simulink model "microgrid"  (R2021b)
settings: Solver=ode23tb  StartTime=0.0  StopTime=1  FixedStep=5e-6  RelTol=1e-3  EnableMultiTasking=on
PreLoadFcn:
  | % ---- microgrid : PreLoadFcn -------------------------------------
  | % Loads every base-workspace parameter this model needs.
  | %   SolarPVMPPTBoostData.mlx : PV array, boost converter, MPPT controller
  | %   microgridParams.m        : bus, battery, grid, drain, droop  (struct mg)
  | try
  |     mgDir = fileparts(which('microgrid'));
  |     if ~isempty(mgDir) && ~contains([path pathsep], [mgDir pathsep])
  |         addpath(mgDir);
  |     end
  |     evalc('SolarPVMPPTBoostData');
  |     microgridParams;
  |     clear mgDir
  |     disp('microgrid: parameters loaded (SolarPVMPPTBoostData + microgridParams).');
  | catch mgErr
  |     warning('microgrid:paramLoadFailed', ...
  |             'Could not load model parameters: %s', mgErr.message);
  |     clear mgErr
  | end
values from neighbouring files (symbols this model uses):
  mg = evalin('base','mg')    [microgridCheck.m]    (also in microgridParams.m = struct(); microgridScenario.m)
undefined symbols (not defined in the file or in its folder): boostController, dcVoltage, Ion, Lithium, sensor, solarPanel, solarPlant
libraries: powerlib_extras x46, fl_lib x12, simulink x8, nesl_utility x8, spsSeriesRLCBranchLib x7, spsCurrentMeasurementLib x7, spsGroundLib x6, spsVoltageMeasurementLib x6, spsIGBTDiodeLib x4, spsVariableResistorLib x4, slpidlib x4, ee_lib x3
(part 1 of 3)
settings Model: Creator=Student  LastModifiedBy=Saad Khan
settings SolverCC: ZeroCrossAlgorithm=Adaptive  AlgebraicLoopSolver=TrustRegion
settings DataIOCC: LimitDataPoints=on  SaveFormat=Array  SignalLoggingSaveFormat=ModelDataLogs  ReturnWorkspaceOutputs=off
settings OptimizationCC: ExpressionDepthLimit=2147483647  LifeSpan=inf
settings DebuggingCC: UnderspecifiedInitializationDetection=Classic  MergeDetectMultiDrivingBlocksExec=none  SolverPrmCheckMsg=warning  FcnCallInpInsideContextMsg=warning  StateNameClashWarn=warning  SFUnexpectedBacktrackingDiag=warning  SFNoUnconditionalDefaultTransitionDiag=warning  SFExecutionAtInitializationDiag=none  ArithmeticOperatorsInVariantConditions=warning
settings HardwareCC: ProdBitPerPointer=32  ProdBitPerSizeT=32  ProdBitPerPtrDiffT=32  ProdLargestAtomicFloat=None  ProdIntDivRoundTo=Undefined  ProdEndianess=Unspecified  ProdWordSize=32  ProdHWDeviceType=32-bit Generic
settings ModelReferenceCC: EnableRefExpFcnMdlSchedulingChecks=off  PropagateSignalLabelsOutOfModel=off
settings SFSimCC: SimUseLocalCustomCode=off  CustomCodeUndefinedFunction=UseInterfaceOnly
settings RTWCC: RTWUseLocalCustomCode=off  DLArmComputeVersion=20.02.1
settings CodeAppCC: StateflowObjectComments=on
settings GRTTargetCC: TargetLangStandard=C89/C90 (ANSI)  CombineOutputUpdateFcns=off  GRTInterface=on
settings ConfigComp: CovMetricSettings=dw  CovSaveCumulativeToWorkspaceVar=on  CovSaveSingleToWorkspaceVar=on  CovExternalEMLEnable=off
settings SimscapeCC: SimscapeNormalizeSystem=off

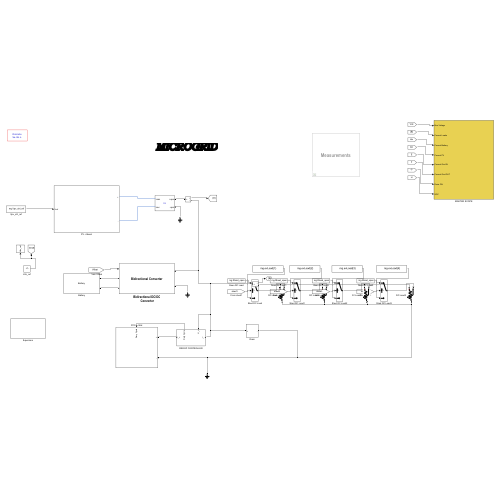
[thumbnail: Simulink's stored preview of the top-level diagram]
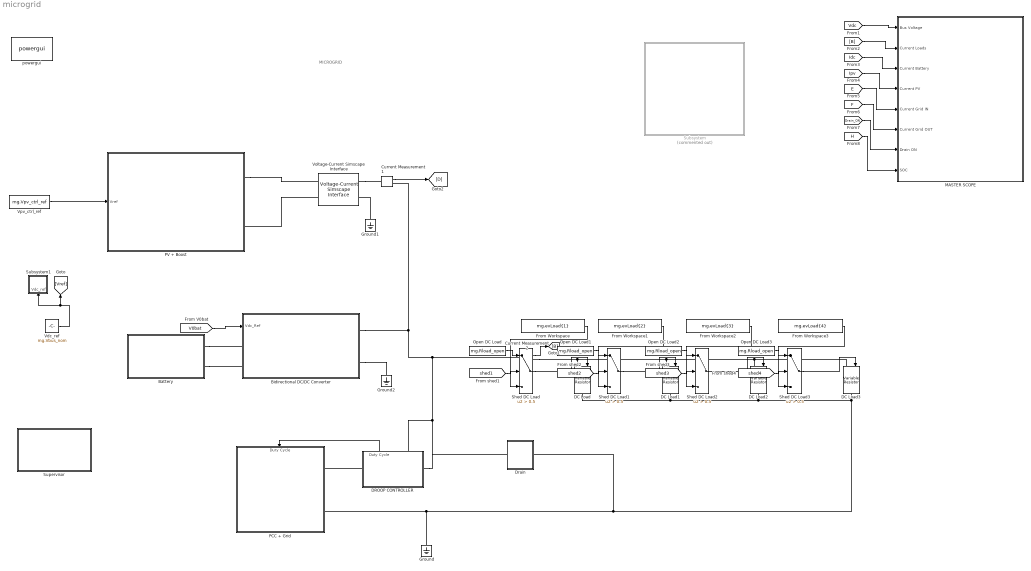
== system microgrid ==
  note: MICROGRID
  Battery : Subsystem
      mask Display:
      | %image(imread('Battery.bmp'))
      | disp('Battery');
  Bidirectional DC/DC Converter : Subsystem
      mask Display: disp('Bidirectional Converter')
  Current Measurement1 : spsCurrentMeasurementLib/Current Measurement  PhasorSimulation=off  OutputType=Complex  PSBequivalent=0
  Current Measurement2 : spsCurrentMeasurementLib/Current Measurement  PhasorSimulation=off  OutputType=Complex  PSBequivalent=0
  DC Load{,1..3} (4 alike) : spsVariableResistorLib/Variable Resistor  Rabsmin=1e-3
      settings: SourceProductBaseCode=PS
  DROOP CONTROLLER : Subsystem
      settings: PortSchema="{\"entries\":[{\"content\":{\"sides\":[{\"content\":{\"connectorIds\":[\"LConn1\"]},\"type\":\"ConnectorPlacement.EquallySpacedRectSide\",\"uuid\":\"2b7abaaf-3c10-498f-b261-e88602c8f41c\"},{\"content\":{\"connectorIds\":[\"RConn1\"],\"side\":\"RIGHT\"},\"type\":\"ConnectorPlacement.EquallySpacedRectSide\",\"uuid\":\"71817c43-ea35-4733-8571-129222f61f00\"},{\"content\":{\"connectorIds\":[\"Out1\",\"LConn2\"],\"side\":\"TOP\"},\"type\":\"ConnectorPlacement.EquallySpacedRectSide\",\"uuid\":\"db48e4ed-dd68-4965-9d82-541b8d604782\"},{\"content\":{\"connectorIds\":[],\"side\":\"BOTTOM\"},\"type\":\"ConnectorPlacement.EquallySpacedRectSide\",\"uuid\":\"50c4439a-898e-4973-8234-14cd96d1453b\"}]},\"type\":\"ConnectorPlacement.EquallySpacedConnector\",\"uuid\":\"1de87e89-706d-458a-94f9-225c5d9d3369\"}],\"packageUris\":[\"http://schema.mathworks.com/mf0/Connector/R2020b\"],\"version\":\"1.0\"}"
  Drain : Subsystem
  From Workspace : FromWorkspace  VariableName=mg.evLoad{1}
  From Workspace1 : FromWorkspace  VariableName=mg.evLoad{2}
  From Workspace2 : FromWorkspace  VariableName=mg.evLoad{3}
  From Workspace3 : FromWorkspace  VariableName=mg.evLoad{4}
  Ground : spsGroundLib/Ground  LConnTagsString=a
  Ground1 : spsGroundLib/Ground  LConnTagsString=a
  Ground2 : spsGroundLib/Ground  LConnTagsString=a
  MASTER SCOPE : Subsystem
  Open DC Load{,1..3} (4 alike) : Constant  Value=mg.Rload_open
  PCC + Grid : Subsystem
      settings: PortSchema="{\"entries\":[{\"content\":{\"sides\":[{\"content\":{\"connectorIds\":[\"LConn1\",\"LConn2\"]},\"type\":\"ConnectorPlacement.EquallySpacedRectSide\",\"uuid\":\"29bea7bc-953f-43d2-87dc-a51f4d1b9249\"},{\"content\":{\"connectorIds\":[],\"side\":\"RIGHT\"},\"type\":\"ConnectorPlacement.EquallySpacedRectSide\",\"uuid\":\"160e404e-4ddb-4454-97d5-9208db6d39a0\"},{\"content\":{\"connectorIds\":[\"In1\"],\"side\":\"TOP\"},\"type\":\"ConnectorPlacement.EquallySpacedRectSide\",\"uuid\":\"154aa630-8823-44c2-b2f2-ecc7273bc090\"}]},\"type\":\"ConnectorPlacement.EquallySpacedConnector\",\"uuid\":\"83e0acdf-9839-4104-a0b3-bfd87becac1e\"}],\"packageUris\":[\"http://schema.mathworks.com/mf0/Connector/R2020b\"],\"version\":\"1.0\"}"
  PV + Boost : Subsystem
  Shed DC Load{,1..3} (4 alike) : Switch  Criteria=u2 > Threshold  Threshold=0.5
  Subsystem : Subsystem  Commented=on
      mask Display: disp('Measurements')
  Subsystem1 : Subsystem
  Supervisor : Subsystem
  Vdc_ref : Constant  Value=mg.Vbus_nom
  Voltage-Current Simscape Interface : spsVoltageCurrentSimscapeInterfaceLib/Voltage-Current Simscape Interface  DFT=off  Fmode=Unit delay (discrete)  T=1e-6  Ts=-1  i0=0  v0=mg.Vbus_nom  Sd=Specialized Power Systems side  Measurements=off
      settings: SourceProductBaseCode=PS
  Vpv_ctrl_ref : Constant  Value=mg.Vpv_ctrl_ref
  powergui : spspowerguiLib/powergui  Priority=1  SimulationMode=Discrete  SampleTime=5e-6  frequency=50  Iterations=50  frequencyindice=0  Pbase=100e6  ErrMax=1e-4  UnitsV=kV  UnitsW=MW  buscounter=0  FunctionMessages=off  echomessages=off  EnableUseOfTLC=off  CurrentSourceSwitches=off  DisableSnubberDevices=off  DisableRonSwitches=off  DisableVfSwitches=off  DisplayEquations=off  AutomaticDiscreteSolvers=off  SolverType=Tustin  Interpol=off  ExternalGateDelay=off  methode=off  Ts=0  x0status=blocks  SPID=off  SwTol=0  HookPort=off  NonlinearTolerance=1e-4  nMaxIteration=100  ContinueOnMaxIteration=off  RestoreLinks=warning  ResistiveCurrentMeasurement=off  Frange=[0:2:500]  Ylog=off  Xlog=on  ShowGrid=off  save=off  variable=ZData  structure=Vab_st  ZoomFFT=off  StartTime=7.5  cycles=4  DisplayStyle=1  fundamental=50  FreqAxis=off  MaxFrequency=50000  frequencyindicesteady=1  RmsSteady=1  display=off
  wires:
  Vdc_ref/1 -> [Vref], Subsystem1/1(Vdc_ref)
  [Vdc] -> MASTER SCOPE/1(Bus Voltage)
  [E] -> MASTER SCOPE/5(Current Grid IN)
  [B] -> MASTER SCOPE/2(Current Loads)
  [Idc] -> MASTER SCOPE/3(Current Battery)
  [Ipv] -> MASTER SCOPE/4(Current PV)
  [F] -> MASTER SCOPE/6(Current Grid OUT)
  [Drain_ON] -> MASTER SCOPE/7(Drain ON)
  [H] -> MASTER SCOPE/8(SOC)
  Current Measurement2/1 -> [B]
  Current Measurement1/1 -> [D]
  DROOP CONTROLLER/1(Duty Cycle) -> PCC + Grid/1(" Dury Cycle ")
  Vpv_ctrl_ref/1 -> PV + Boost/1(Vref)
  [V0bat] -> Bidirectional DC/DC Converter/1(Vdc_Ref)
  Open DC Load/1 -> Shed DC Load/1
  [shed1] -> Shed DC Load/2
  From Workspace/1 -> Shed DC Load/3
  Shed DC Load/1 -> DC Load/1
  Open DC Load1/1 -> Shed DC Load1/1
  [shed2] -> Shed DC Load1/2
  From Workspace1/1 -> Shed DC Load1/3
  Shed DC Load1/1 -> DC Load1/1
  Open DC Load2/1 -> Shed DC Load2/1
  [shed3] -> Shed DC Load2/2
  From Workspace2/1 -> Shed DC Load2/3
  Shed DC Load2/1 -> DC Load2/1
  Open DC Load3/1 -> Shed DC Load3/1
  [shed4] -> Shed DC Load3/2
  From Workspace3/1 -> Shed DC Load3/3
  Shed DC Load3/1 -> DC Load3/1
  connections:
  Battery/LConn1 -- Bidirectional DC/DC Converter/LConn1
  Battery/LConn2 -- Bidirectional DC/DC Converter/LConn2
  Voltage-Current Simscape Interface/RConn2 -- PV + Boost/RConn2
  PV + Boost/RConn1 -- Voltage-Current Simscape Interface/RConn1
  Current Measurement2/LConn1 -- DROOP CONTROLLER/RConn1 -- Drain/LConn1 -- DROOP CONTROLLER/LConn2 -- Bidirectional DC/DC Converter/RConn1 -- Current Measurement1/RConn1
  DC Load3/LConn1 -- Current Measurement2/RConn1 -- DC Load/LConn1 -- DC Load1/LConn1 -- DC Load2/LConn1
  DC Load2/RConn1 -- Drain/RConn1 -- PCC + Grid/LConn2 -- Ground/LConn1 -- DC Load3/RConn1 -- DC Load/RConn1 -- DC Load1/RConn1
  Ground1/LConn1 -- Voltage-Current Simscape Interface/LConn2
  DROOP CONTROLLER/LConn1 -- PCC + Grid/LConn1
  Voltage-Current Simscape Interface/LConn1 -- Current Measurement1/LConn1
  Bidirectional DC/DC Converter/RConn2 -- Ground2/LConn1

== system microgrid/Battery ==
  Battery : spsBatteryLib/Battery  BatType=Lithium-Ion  ShowTempParam=off  ThermalPreset=no  ShowAgeParam=off  NomV=mg.Vbat_nom  NomQ=mg.Qbat_Ah  SOC=mg.SOC0  Batt_Tr=1  PresetModel=on  MaxQ=600  MinV=300  FullV=465.5949  Dis_rate=260.8696  R=0.0066667  Normal_OP=542.6087  expZone="[432.1543      29.47826]"  current=[1.3 2.6 6.5]  Units=Time  Tci=20  NomT=20  T2=-30  MaxQ2=4.8  FullV2=7.1  Normal_OP2=5.655  expZone2="[6.58           1]"  Rca=0.6  ti=2000  Dp=0  Neq0=0  Tsim=1e6  Ta1=25  Qeol=5.4*0.9  Reol=0.013333*1.2  Char_age=[2.3478, 3]  Dis_age=[2.3478, 10]  N1=1500  N2=10500  N3=1000  N4=1400  Ta2=45  N5=950
  Bus Selector : BusSelector  OutputSignals=SOC (%),Current (A),Voltage (V)
  Ground : spsGroundLib/Ground  LConnTagsString=a
  LPF vq1 : powerlib_extras/Discrete  Control Blocks/Discrete 1st-Order Filter  FilterType=Lowpass  Tc=10e-3  Ts=5e-6  Initialize=off  Vac_Init=[0.8 -25 60]  Vdc_Init=0  PlotResponse=off  param1=[1 100 0.1]
      settings: SourceProductBaseCode=PS
  LPF vq2 : powerlib_extras/Discrete  Control Blocks/Discrete 1st-Order Filter  FilterType=Lowpass  Tc=10e-3  Ts=5e-6  Initialize=off  Vac_Init=[0.8 -25 60]  Vdc_Init=0  PlotResponse=off  param1=[1 100 0.1]
      settings: SourceProductBaseCode=PS
  SOC : Scope
  Subsystem1 : Subsystem
  Subsystem2 : Subsystem
  Subsystem5 : Subsystem
  Vbat : Scope
  + : PMIOPort  Side=Left
  - : PMIOPort  Port=2  Side=Left
  tag scope: H=global
  wires:
  Battery/1 -> Bus Selector/1
  Bus Selector/2 -> LPF vq1/1  "<Current (A)>"
  LPF vq1/1 -> Subsystem1/1(Ibat)
  Bus Selector/1 -> [H], SOC/1, Subsystem5/1(SOC)  "<SOC (%)>"
  Bus Selector/3 -> Vbat/1, LPF vq2/1  "<Voltage (V)>"
  LPF vq2/1 -> Subsystem2/1(Vbat)
  connections:
  -/RConn1 -- Ground/LConn1 -- Battery/LConn2
  Battery/LConn1 -- +/RConn1

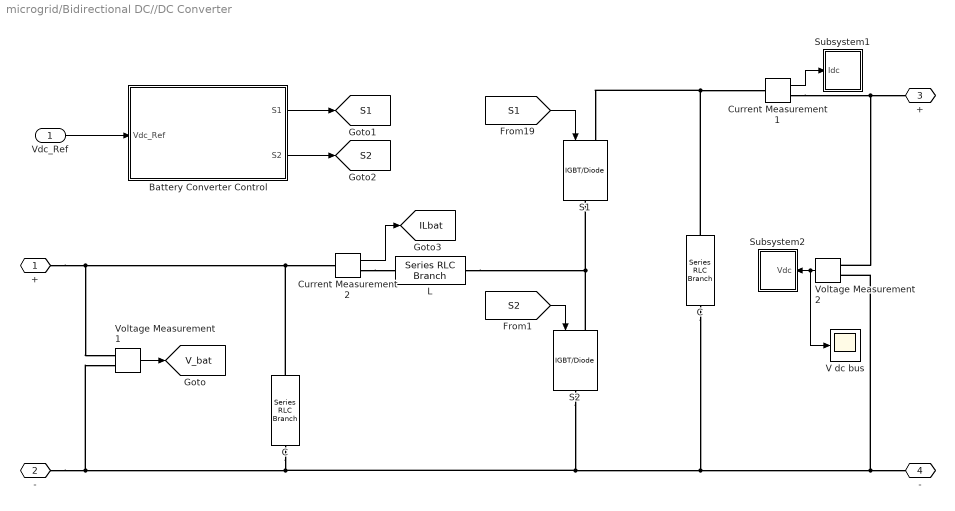
== system microgrid/Bidirectional DC//DC Converter ==
  Vdc_Ref : Inport
  Battery Converter Control : Subsystem
  C : spsSeriesRLCBranchLib/Series RLC Branch  LConnTagsString=__new0  RConnTagsString=__new0  BranchType=RC  Resistance=0.01  Inductance=1e-3  SetiL0=off  InitialCurrent=0  Capacitance=mg.Cbat_bus  Setx0=on  InitialVoltage=mg.Vbus_nom  Measurements=None
  "C " : spsSeriesRLCBranchLib/Series RLC Branch  LConnTagsString=__new0  RConnTagsString=__new0  BranchType=RC  Resistance=0.01  Inductance=1e-3  SetiL0=off  InitialCurrent=0  Capacitance=mg.Cbat  Setx0=on  InitialVoltage=mg.Vbat_C0  Measurements=None
  Current Measurement1 : spsCurrentMeasurementLib/Current Measurement  PhasorSimulation=off  OutputType=Complex  PSBequivalent=0
  Current Measurement2 : spsCurrentMeasurementLib/Current Measurement  PhasorSimulation=off  OutputType=Complex  PSBequivalent=0
  L : spsSeriesRLCBranchLib/Series RLC Branch  LConnTagsString=__new0  RConnTagsString=__new0  BranchType=L  Resistance=mg.Rbat_L  Inductance=mg.Lbat  SetiL0=on  InitialCurrent=0  Capacitance=1e-6  Setx0=off  InitialVoltage=0  Measurements=None
  "S1 " : spsIGBTDiodeLib/IGBT//Diode  Ron=mg.Ron  Rs=mg.Rsnub  Cs=inf  Measurements=off
  "S2 " : spsIGBTDiodeLib/IGBT//Diode  Ron=mg.Ron  Rs=mg.Rsnub  Cs=inf  Measurements=off
  Subsystem1 : Subsystem
  Subsystem2 : Subsystem
  V dc bus : Scope
  Voltage Measurement1 : spsVoltageMeasurementLib/Voltage Measurement  PhasorSimulation=off  OutputType=Complex  PSBequivalent=0
  Voltage Measurement2 : spsVoltageMeasurementLib/Voltage Measurement  PhasorSimulation=off  OutputType=Complex  PSBequivalent=0
  "+ " : PMIOPort  Side=Left
  "-  " : PMIOPort  Port=2  Side=Left
  + : PMIOPort  Port=3  Side=Right
  - : PMIOPort  Port=4  Side=Right
  tag scope: ILbat=global, S1=global, S2=global, V_bat=global
  wires:
  Voltage Measurement1/1 -> [V_bat]
  Current Measurement2/1 -> [ILbat]
  Battery Converter Control/1(S1) -> [S1]
  Battery Converter Control/2(S2) -> [S2]
  [S1] -> "S1 "/1
  [S2] -> "S2 "/1
  Voltage Measurement2/1 -> V dc bus/1, Subsystem2/1(Vdc)
  Current Measurement1/1 -> Subsystem1/1(Idc)
  Vdc_Ref/1 -> Battery Converter Control/1(Vdc_Ref)
  connections:
  "-  "/RConn1 -- Voltage Measurement1/LConn2 -- "C "/RConn1 -- "S2 "/RConn1 -- C/RConn1 -- -/RConn1 -- Voltage Measurement2/LConn2
  "S2 "/LConn1 -- "S1 "/RConn1 -- L/RConn1
  C/LConn1 -- "S1 "/LConn1 -- Current Measurement1/LConn1
  Current Measurement2/RConn1 -- L/LConn1
  "+ "/RConn1 -- Voltage Measurement1/LConn1 -- "C "/LConn1 -- Current Measurement2/LConn1
  Current Measurement1/RConn1 -- +/RConn1 -- Voltage Measurement2/LConn1

== system microgrid/DROOP CONTROLLER ==
  Current Measurement : spsCurrentMeasurementLib/Current Measurement  PhasorSimulation=off  OutputType=Complex  PSBequivalent=0
  Grid Droop : microgridLib/DC Droop Node  Rdroop=mg.Rdroop_grid  DB=mg.DB_grid  Tf=mg.Tf_droop  Imin=mg.Igrid_min  Imax=mg.Igrid_max  Vinit=mg.Vbus_nom
  Ground : spsGroundLib/Ground  LConnTagsString=a
  Igrid limit : simulink/Discontinuities/Saturation Dynamic  OutMin=[]  OutMax=[]  OutDataTypeStr=Inherit: Same as second input  OutDataType=fixdt(1, 16)  OutScaling=2^-10  DoSatur=off
  PID Controller : slpidlib/PID Controller  Controller=PI  Form=Parallel  TimeDomain=Continuous-time  UseExternalTs=off  SampleTime=-1  IntegratorMethod=Forward Euler  FilterMethod=Forward Euler  ControllerParametersSource=internal  P=mg.Kp_i_gdc  I=mg.Ki_i_gdc  D=0  UseFilter=on  N=100  TunerSelectOption=Transfer Function Based (PID Tuner App)  InitialConditionSource=internal  InitialConditionForIntegrator=mg.Dgdc_nom  InitialConditionForFilter=0  DifferentiatorICPrevScaledInput=0  ExternalReset=none  TrackingMode=off  Kt=1  LimitOutput=on  SatLimitsSource=internal  UpperSaturationLimit=1  LowerSaturationLimit=0  LinearizeAsGain=on  AntiWindupMode=clamping  Kb=1  POutMin=[]  POutMax=[]  IOutMin=[]  IOutMax=[]  DOutMin=[]  DOutMax=[]  NOutMin=[]  NOutMax=[]  SumOutMin=[]  SumOutMax=[]  SaturationOutMin=[]  SaturationOutMax=[]  PParamMin=[]  PParamMax=[]  IParamMin=[]  IParamMax=[]  DParamMin=[]  DParamMax=[]  NParamMin=[]  NParamMax=[]  KbParamMin=[]  KbParamMax=[]  KtParamMin=[]  KtParamMax=[]  KbOutMin=[]  KbOutMax=[]  KtOutMin=[]  KtOutMax=[]  IntegratorOutMin=[]  IntegratorOutMax=[]  FilterOutMin=[]  FilterOutMax=[]  SumI1OutMin=[]  SumI1OutMax=[]  SumI2OutMin=[]  SumI2OutMax=[]  SumI3OutMin=[]  SumI3OutMax=[]  SumI4OutMin=[]  SumI4OutMax=[]  SumDOutMin=[]  SumDOutMax=[]  DifferentiatorOutMin=[]  DifferentiatorOutMax=[]  FilterDiffOutCoefMin=[]  FilterDiffOutCoefMax=[]  ReciprocalOutMin=[]  ReciprocalOutMax=[]  SumDenOutMin=[]  SumDenOutMax=[]  SumNumOutMin=[]  SumNumOutMax=[]  DivideOutMin=[]  DivideOutMax=[]  UdiffTsProdOutMin=[]  UdiffTsProdOutMax=[]  NTsProdOutMin=[]  NTsProdOutMax=[]  UintegralTsProdOutMin=[]  UintegralTsProdOutMax=[]  UngainTsProdOutMin=[]  UngainTsProdOutMax=[]  FilterDenConstantOutDataTypeStr=Inherit: Inherit via back propagation  FilterDenConstantOutMin=[]  FilterDenConstantOutMax=[]  PCopyOutDataTypeStr=Inherit: Inherit via back propagation  PCopyOutMin=[]  PCopyOutMax=[]  NCopyOutDataTypeStr=Inherit: Inherit via back propagation  NCopyOutMin=[]  NCopyOutMax=[]  IntegratorContinuousStateAttributes=''  IntegratorStateMustResolveToSignalObject=off  IntegratorRTWStateStorageClass=Auto  FilterContinuousStateAttributes=''  FilterStateMustResolveToSignalObject=off  FilterRTWStateStorageClass=Auto  ParallelPVariant=InternalParameters  IdealPVariant=Disabled  IVariant=InternalParameters  DVariant=Disabled  IntegratorVariant=Continuous  SatVariant=Enabled  AWVariant=ContClampingParallel  PCopyVariant=Disabled  TRVariant=Disabled  FdbkBlocksVariant=Forward  IdealPFdbkVariant=Disabled  SatFdbkVariant=Disabled  DerivativeFilterVariant=Disabled  NVariant=Disabled  NCopyVariant=Disabled_SignalSpec  FilterICVariant=Disabled  IntegratorICVariant=InternalICs  ExternalResetVariant=Disabled  TRSumVariant=Passthrough  SumFdbkVariant=Disabled  SumVariant=Sum_PI  TsampFilterVariant=InternalTs  TsampNgainVariant=Passthrough  TsampIntegralVariant=Passthrough  ExternalSaturationOutDataTypeStr=Inherit: Same as second input
  Subtract1 : Sum  Inputs=+-
  Voltage Measurement : spsVoltageMeasurementLib/Voltage Measurement  PhasorSimulation=off  OutputType=Complex  PSBequivalent=0
  log Igrid ref : ToWorkspace  VariableName=Igrid_ref  SampleTime=-1
      settings: Decimation=20
  I_+ : PMIOPort  Side=Left
  U_+ : PMIOPort  Port=2  Side=Left
  I_- : PMIOPort  Port=3  Side=Right
  Duty Cycle : Outport
  tag scope: F=global
  wires:
  Subtract1/1 -> PID Controller/1
  PID Controller/1 -> [F], Duty Cycle/1
  Current Measurement/1 -> Subtract1/2
  [V0grid] -> Grid Droop/1
  Voltage Measurement/1 -> Grid Droop/2
  [Igrid_hi] -> Igrid limit/1
  Grid Droop/1 -> Igrid limit/2
  [Igrid_lo] -> Igrid limit/3
  Igrid limit/1 -> Subtract1/1, log Igrid ref/1
  connections:
  I_-/RConn1 -- Current Measurement/RConn1
  Voltage Measurement/LConn1 -- U_+/RConn1
  I_+/RConn1 -- Current Measurement/LConn1
  Ground/LConn1 -- Voltage Measurement/LConn2

== system microgrid/Drain ==
  Current Measurement1 : spsCurrentMeasurementLib/Current Measurement  PhasorSimulation=off  OutputType=Complex  PSBequivalent=0
  Drain hysteresis : Relay  OnSwitchValue=mg.Vdrain_on  OffSwitchValue=mg.Vdrain_off
  Ground : spsGroundLib/Ground  LConnTagsString=a
  Ideal Switch : spsIdealSwitchLib/Ideal Switch  Ron=mg.Rdrain_on  Lon=0  IC=0  Rs=9999999  Cs=inf  Measurements=off
  Idrain filt term : Terminator
  Series RLC Branch : spsSeriesRLCBranchLib/Series RLC Branch  LConnTagsString=__new0  RConnTagsString=__new0  BranchType=R  Resistance=mg.Rdrain  Inductance=1e-3  SetiL0=off  InitialCurrent=0  Capacitance=1e-6  Setx0=off  InitialVoltage=0  Measurements=None
  Transfer Fcn : TransferFcn  Denominator=[1 1]
  Voltage Measurement : spsVoltageMeasurementLib/Voltage Measurement  PhasorSimulation=off  OutputType=Complex  PSBequivalent=0
  + : PMIOPort  Side=Left
  - : PMIOPort  Port=2  Side=Right
  tag scope: Drain_ON=global
  wires:
  Current Measurement1/1 -> Transfer Fcn/1
  Transfer Fcn/1 -> Idrain filt term/1
  Voltage Measurement/1 -> Drain hysteresis/1
  Drain hysteresis/1 -> Ideal Switch/1, [Drain_ON]
  connections:
  Ideal Switch/LConn1 -- Voltage Measurement/LConn1 -- +/RConn1
  Series RLC Branch/RConn1 -- -/RConn1
  Ground/LConn1 -- Voltage Measurement/LConn2
  Current Measurement1/LConn1 -- Ideal Switch/RConn1
  Current Measurement1/RConn1 -- Series RLC Branch/LConn1

== system microgrid/MASTER SCOPE ==
  Bus Voltage : Inport
  Current Loads : Inport  Port=2
  Current Battery : Inport  Port=3
  Current PV : Inport  Port=4
  Current Grid IN : Inport  Port=5
  Current Grid OUT : Inport  Port=6
  Drain ON : Inport  Port=7
  SOC : Inport  Port=8
  MASTER SCOPE : Scope  NumInputPorts=8
  wires:
  Bus Voltage/1 -> MASTER SCOPE/1
  Current Loads/1 -> MASTER SCOPE/2
  Current Battery/1 -> MASTER SCOPE/3
  Current PV/1 -> MASTER SCOPE/4
  Current Grid IN/1 -> MASTER SCOPE/5
  Current Grid OUT/1 -> MASTER SCOPE/6
  Drain ON/1 -> MASTER SCOPE/7
  SOC/1 -> MASTER SCOPE/8

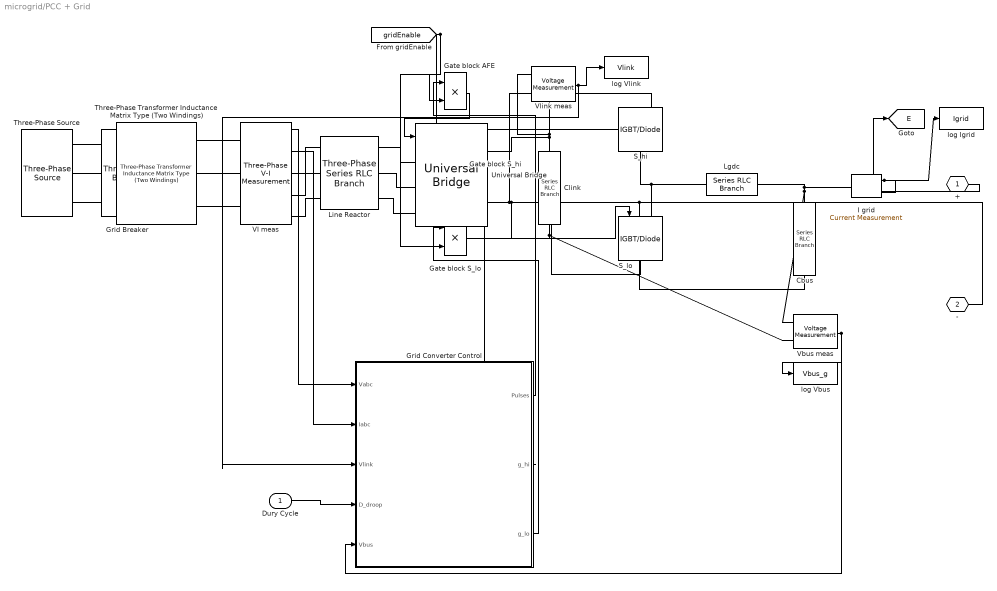
== system microgrid/PCC + Grid ==
  " Dury Cycle " : Inport
  Cbus : spsSeriesRLCBranchLib/Series RLC Branch  LConnTagsString=__new0  RConnTagsString=__new0  BranchType=RC  Resistance=mg.Resr  Inductance=1e-3  SetiL0=off  InitialCurrent=0  Capacitance=mg.Cgdc_bus  Setx0=on  InitialVoltage=mg.Vbus_nom  Measurements=None
  Clink : spsSeriesRLCBranchLib/Series RLC Branch  LConnTagsString=__new0  RConnTagsString=__new0  BranchType=C  Resistance=1  Inductance=1e-3  SetiL0=off  InitialCurrent=0  Capacitance=mg.Clink  Setx0=on  InitialVoltage=mg.Vlink_ref  Measurements=None
  Gate block AFE : Product
  Gate block S_hi : Product
  Gate block S_lo : Product
  Grid Breaker : spsThreePhaseBreakerLib/Three-Phase Breaker  InitialState=closed  SwitchA=on  SwitchB=on  SwitchC=on  SwitchTimes=[mg.t_island mg.t_reconnect]  External=off  BreakerResistance=mg.Ron  SnubberResistance=mg.Rsnub  SnubberCapacitance=inf  Measurements=None
  Grid Converter Control : Subsystem
  I grid : spsCurrentMeasurementLib/Current Measurement  PhasorSimulation=off  OutputType=Complex  PSBequivalent=0
  Lgdc : spsSeriesRLCBranchLib/Series RLC Branch  LConnTagsString=__new0  RConnTagsString=__new0  BranchType=L  Resistance=mg.Rgdc  Inductance=mg.Lgdc  SetiL0=off  InitialCurrent=0  Capacitance=1e-6  Setx0=off  InitialVoltage=0  Measurements=None
  Line Reactor : spsThreePhaseSeriesRLCBranchLib/Three-Phase Series RLC Branch  LConnTagsString=A|B|C  RConnTagsString=A|B|C  BranchType=RL  Resistance=mg.Rgrid  Inductance=mg.Lgrid  Capacitance=1e-6  Measurements=None
  S_hi : spsIGBTDiodeLib/IGBT//Diode  Ron=mg.Ron  Rs=mg.Rsnub  Cs=mg.Csnub  Measurements=off
  S_lo : spsIGBTDiodeLib/IGBT//Diode  Ron=mg.Ron  Rs=mg.Rsnub  Cs=mg.Csnub  Measurements=off
  Three-Phase Source : spsThreePhaseSourceLib/Three-Phase Source  InternalConnection=Yg  VoltagePhases=off  Voltage=mg.Vgrid_LL  PhaseAngle=0  Voltage_phases=[25e3 25e3 25e3]/sqrt(3)  PhaseAngles_phases=[0 -120 +120]  Frequency=mg.fgrid  NonIdealSource=on  SpecifyImpedance=off  Resistance=0.8929  Inductance=16.58e-3  ShortCircuitLevel=100e6  BaseVoltage=25e3  XRratio=7  BusType=swing  Pref=10e3  Qref=0  Prefabc=[10e3, 10e3, 10e3]  Qrefabc=[0, 0, 0]  Qmin=-inf  Qmax=inf
  Three-Phase Transformer Inductance Matrix Type (Two Windings) : spsThreePhaseTransformerInductanceMatrixTypeTwoWindingsLib/Three-Phase Transformer Inductance Matrix Type (Two Windings)  CoreType=Three-limb or five-limb core  Winding1Connection=Yg  Winding2Connection=Y  AutoTransformer=off  Measurements=None  NominalPower=[800e3, 50]  VLLnom=[25000, 800]  WindingResistances=[0.01, 0.01]  NoLoadIexcPos=2  NoLoadPlossPos=1000  ShortCircuitReactancePos=0.06  ShortCircuitReactancePosAuto=0.06  NoLoadIexcZero=2  NoLoadPlossZero=1500  ShortCircuitReactanceZero=0.03  ShortCircuitReactanceZeroAuto=0.03
      settings: SourceProductBaseCode=PS
  Universal Bridge : spsUniversalBridgeLib/Universal Bridge  Arms=3  SnubberResistance=mg.Rsnub  SnubberCapacitance=mg.Csnub  Device=IGBT / Diodes  Ron=mg.Ron  Lon=0  ForwardVoltages="[  0  0  ]"  ForwardVoltage=0  GTOparameters=[ 10e-6 , 20e-6 ]  IGBTparameters=[ 1e-6 , 2e-6 ]  Measurements=None  Measurements_2=None  converterType=Rectifier
  VI meas : spsThreePhaseVIMeasurementLib/Three-Phase V-I Measurement  VoltageMeasurement=phase-to-ground  SetLabelV=off  LabelV=Vabc  Vpu=off  VpuLL=off  CurrentMeasurement=yes  SetLabelI=off  LabelI=Iabc  Ipu=off  Pbase=100e6  Vbase=500e3  OutputType=Complex  PhasorSimulation=off  PSBequivalent=0
  Vbus meas : spsVoltageMeasurementLib/Voltage Measurement  PhasorSimulation=off  OutputType=Complex  PSBequivalent=0
  Vlink meas : spsVoltageMeasurementLib/Voltage Measurement  PhasorSimulation=off  OutputType=Complex  PSBequivalent=0
  log Igrid : ToWorkspace  VariableName=Igrid  SampleTime=-1
      settings: Decimation=20
  log Vbus : ToWorkspace  VariableName=Vbus_g  SampleTime=-1
      settings: Decimation=20
  log Vlink : ToWorkspace  VariableName=Vlink  SampleTime=-1
      settings: Decimation=20
  + : PMIOPort  Side=Left
  - : PMIOPort  Port=2  Side=Left
  tag scope: E=global
  wires:
  I grid/1 -> [E], log Igrid/1
  VI meas/1 -> Grid Converter Control/1(Vabc)
  VI meas/2 -> Grid Converter Control/2(Iabc)
  Vlink meas/1 -> Grid Converter Control/3(Vlink), log Vlink/1
  " Dury Cycle "/1 -> Grid Converter Control/4(D_droop)
  Vbus meas/1 -> Grid Converter Control/5(Vbus), log Vbus/1
  Grid Converter Control/1(Pulses) -> Gate block AFE/1
  [gridEnable] -> Gate block AFE/2, Gate block S_hi/2, Gate block S_lo/2
  Gate block AFE/1 -> Universal Bridge/1
  Grid Converter Control/2(g_hi) -> Gate block S_hi/1
  Gate block S_hi/1 -> S_hi/1
  Grid Converter Control/3(g_lo) -> Gate block S_lo/1
  Gate block S_lo/1 -> S_lo/1
  connections:
  Three-Phase Transformer Inductance Matrix Type (Two Windings)/RConn1 -- VI meas/LConn1
  Three-Phase Transformer Inductance Matrix Type (Two Windings)/RConn2 -- VI meas/LConn2
  Three-Phase Transformer Inductance Matrix Type (Two Windings)/RConn3 -- VI meas/LConn3
  VI meas/RConn1 -- Line Reactor/LConn1
  VI meas/RConn2 -- Line Reactor/LConn2
  VI meas/RConn3 -- Line Reactor/LConn3
  Line Reactor/RConn1 -- Universal Bridge/LConn1
  Line Reactor/RConn2 -- Universal Bridge/LConn2
  Line Reactor/RConn3 -- Universal Bridge/LConn3
  Universal Bridge/RConn1 -- S_hi/LConn1 -- Vlink meas/LConn1 -- Clink/LConn1
  Universal Bridge/RConn2 -- -/RConn1 -- Cbus/RConn1 -- S_lo/RConn1 -- Clink/RConn1 -- Vbus meas/LConn2 -- Vlink meas/LConn2
  S_lo/LConn1 -- S_hi/RConn1 -- Lgdc/LConn1
  Lgdc/RConn1 -- I grid/LConn1 -- Cbus/LConn1 -- Vbus meas/LConn1
  I grid/RConn1 -- +/RConn1
  Three-Phase Source/RConn1 -- Grid Breaker/LConn1
  Grid Breaker/RConn1 -- Three-Phase Transformer Inductance Matrix Type (Two Windings)/LConn1
  Three-Phase Source/RConn2 -- Grid Breaker/LConn2
  Grid Breaker/RConn2 -- Three-Phase Transformer Inductance Matrix Type (Two Windings)/LConn2
  Three-Phase Source/RConn3 -- Grid Breaker/LConn3
  Grid Breaker/RConn3 -- Three-Phase Transformer Inductance Matrix Type (Two Windings)/LConn3

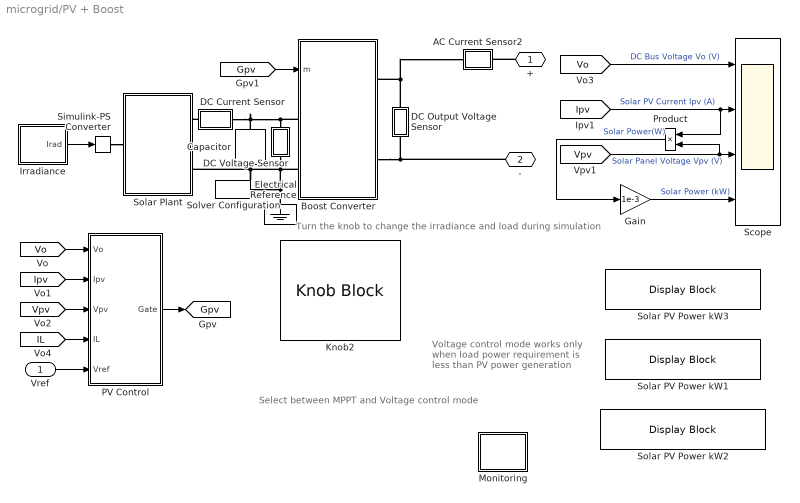
== system microgrid/PV + Boost ==
  note: Voltage control mode works only when load power requirement is less than PV power generation
  note: Select between MPPT and Voltage control mode
  note: Turn the knob to change the irradiance and load during simulation
  Vref : Inport
  AC Current Sensor2 : Subsystem
      mask Display: disp('i');
  Boost Converter : Subsystem  VariantControl=boostCircuit == 1
  Capacitor : fl_lib/Electrical/Electrical Elements/Capacitor  c=boost.inputCapacitor F  r=1e-6 Ohm  g=0 1/Ohm  i_specify=off  i_priority=None  i=0 A  i_nominal_specify=off  i_nominal_unit=A  i_nominal_value=1  v_specify=off  v_priority=None  v=solarPlant.startMPPTValue V  v_nominal_specify=off  v_nominal_unit=V  v_nominal_value=1  vc_specify=on  vc_priority=High  vc=solarPlant.startMPPTValue V  vc_nominal_specify=off  vc_nominal_unit=V  vc_nominal_value=1
  DC Current Sensor : Subsystem
      mask Display: disp('i')
  DC Output Voltage Sensor : Subsystem
      mask Display: disp('v')
  DC Voltage Sensor : Subsystem
      mask Display: disp('v');
  Electrical Reference : fl_lib/Electrical/Electrical Elements/Electrical Reference
  Gain : Gain  Gain=1e-3
  Irradiance : Subsystem
  Knob2 : KnobBlock  ScaleMin=150  ScaleMax=1000
  Monitoring : Subsystem
  PV Control : Subsystem
  Product : Product
  Scope : Scope  NumInputPorts=4
  Simulink-PS Converter : nesl_utility/Simulink-PS Converter  PhysicalDomain=network_engine_domain  SubClassName=ps_input  LeftPortType=input  RightPortType=output  PseudoPeriodic=off  Frequencies=[]  NoiseDistribution=none  NoiseParameters=[]  Unit=1  AffineConversion=off  FilteringAndDerivatives=provide  SimscapeFilterOrder=1  InputFilterTimeConstant=0.001  UdotUserProvided=0
      settings: SourceProductBaseCode=PW,SS
  Solar PV Power kW1 : DisplayBlock  Format=short  Transparency=1
  Solar PV Power kW2 : DisplayBlock  Format=short  Transparency=1
  Solar PV Power kW3 : DisplayBlock  Format=short  Transparency=1
  Solar Plant : Subsystem
  Solver Configuration : nesl_utility/Solver Configuration  PhysicalDomain=network_engine_domain  SubClassName=solver  LeftPortType=input  RightPortType=generic  Tones=[]  Harmonics=[]  SimulateNoise=off  Profile=off  UseLocalSampling=off  EnableSwitchedLinearOptims=on  FrequencyDomain=off  UseCCode=off  RelTol=0.001  AbsTol=1e-06  MinStep=1e-09  ToWorkspace=off  RevertToSquareIcSolve=off  NumHomotopyIterations=100  PhasorMode=off  PhasorModeNumHarmonics=1  DoDC=off  ResidualTolerance=1e-9  UseLocalSolver=off  LocalSolverChoice=NE_BACKWARD_EULER_ADVANCER  LocalSolverSampleTime=1e-6  DoFixedCost=off  MaxNonlinIter=10  MaxModeIter=2  ComputeImpulses=off  ImpulseIterations=2  LinearAlgebra=auto  EquationFormulation=NE_TIME_EF  DelaysMemoryBudget=1024  AutomaticFiltering=on  FilteringTimeConstant=0.001  PartitionStorageMethod=AS_NEEDED  PartitionMemoryBudget=1024  PartitionMethod=FAST
      settings: SourceProductBaseCode=PW,SS
  + : PMIOPort  Side=Right
  - : PMIOPort  Port=2  Side=Right
  tag scope: Gpv=global
  wires:
  [IL] -> PV Control/4(IL)
  Irradiance/1(Irad) -> Simulink-PS Converter/1
  [Ipv] -> PV Control/2(Ipv)
  [Ipv] -> Product/1, Scope/2  "Solar PV Current Ipv (A)"
  PV Control/1(Gate) -> [Gpv]
  [Vo] -> PV Control/1(Vo)
  [Vpv] -> Product/2, Scope/3  "Solar Panel Voltage Vpv (V)"
  [Vpv] -> PV Control/3(Vpv)
  Product/1 -> Gain/1  "Solar Power(W)"
  [Vo] -> Scope/1  "DC Bus Voltage Vo (V)"
  [Gpv] -> Boost Converter/1(m)
  Gain/1 -> Scope/4  "Solar Power (kW)"
  Vref/1 -> PV Control/5(Vref)
  connections:
  Electrical Reference/LConn1 -- Solar Plant/RConn2 -- Capacitor/RConn1 -- Boost Converter/LConn2 -- DC Voltage Sensor/LConn1 -- Solver Configuration/RConn1
  Boost Converter/LConn1 -- DC Voltage Sensor/RConn1 -- DC Current Sensor/LConn1 -- Capacitor/LConn1
  DC Current Sensor/RConn1 -- Solar Plant/RConn1
  Boost Converter/RConn2 -- -/RConn1 -- DC Output Voltage Sensor/LConn1
  Simulink-PS Converter/RConn1 -- Solar Plant/LConn1
  +/RConn1 -- AC Current Sensor2/LConn1
  Boost Converter/RConn1 -- DC Output Voltage Sensor/RConn1 -- AC Current Sensor2/RConn1

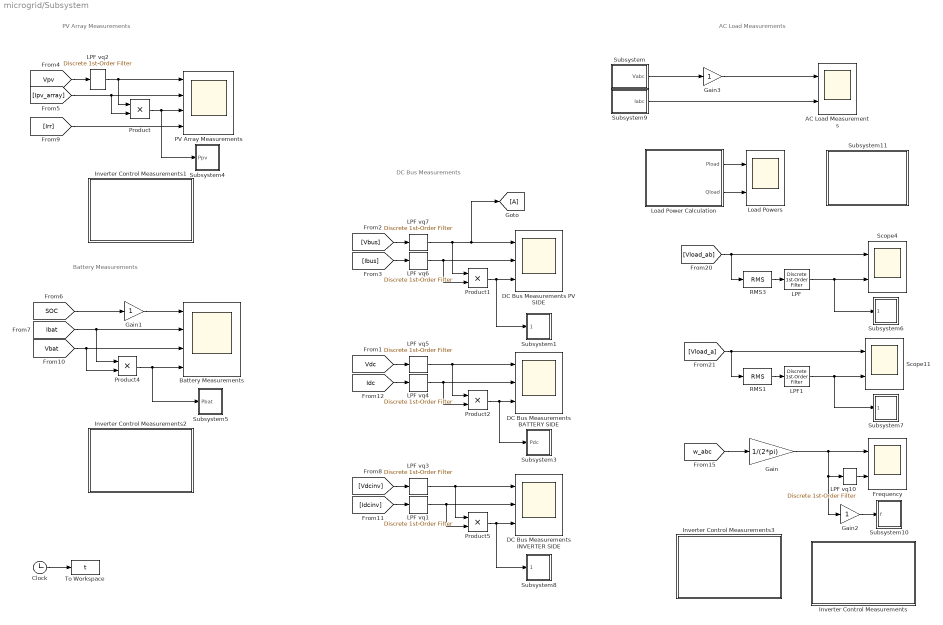
== system microgrid/Subsystem ==
  note: PV Array Measurements
  note: Battery Measurements
  note: DC Bus Measurements
  note: AC Load Measurements
  AC Load Measurements : Scope  NumInputPorts=2
  Battery Measurements : Scope  NumInputPorts=4
  Clock : Clock
  DC Bus Measurements BATTERY SIDE : Scope  NumInputPorts=3
  DC Bus Measurements INVERTER SIDE : Scope  NumInputPorts=3
  DC Bus Measurements PV SIDE : Scope  NumInputPorts=3
  Frequency : Scope  NumInputPorts=2
  Gain : Gain  Gain=1/(2*pi)
  Gain1 : Gain
  Gain2 : Gain
  Gain3 : Gain
  Inverter Control Measurements : Subsystem
      mask Display: disp('Inverter Control')
  Inverter Control Measurements1 : Subsystem
      mask Display: disp('Boost Converter Control')
  Inverter Control Measurements2 : Subsystem
      mask Display: disp('Bidirectional Converter Control')
  Inverter Control Measurements3 : Subsystem
      mask Display: disp('Frequency Measurement')
  LPF : powerlib_extras/Discrete  Control Blocks/Discrete 1st-Order Filter  FilterType=Lowpass  Tc=10e-3  Ts=5e-6  Initialize=off  Vac_Init=[0.8 -25 60]  Vdc_Init=0  PlotResponse=off  param1=[1 100 0.1]
      settings: SourceProductBaseCode=PS
  LPF vq{1..7,10} (8 alike) : powerlib_extras/Discrete  Control Blocks/Discrete 1st-Order Filter  FilterType=Lowpass  Tc=10e-3  Ts=5e-6  Initialize=off  Vac_Init=[0.8 -25 60]  Vdc_Init=0  PlotResponse=off  param1=[1 100 0.1]
      settings: SourceProductBaseCode=PS
  LPF1 : powerlib_extras/Discrete  Control Blocks/Discrete 1st-Order Filter  FilterType=Lowpass  Tc=10e-3  Ts=5e-6  Initialize=off  Vac_Init=[0.8 -25 60]  Vdc_Init=0  PlotResponse=off  param1=[1 100 0.1]
      settings: SourceProductBaseCode=PS
  Load Power Calculation : Subsystem
  Load Powers : Scope  NumInputPorts=2
  PV Array Measurements : Scope  NumInputPorts=4
  Product{,1..2,4..5} (5 alike) : Product  RndMeth=Zero
  RMS1 : powerlib_extras/Measurements/RMS  f1=60
      settings: SourceProductBaseCode=PS
  RMS3 : powerlib_extras/Measurements/RMS  f1=60
      settings: SourceProductBaseCode=PS
  Scope11 : Scope  NumInputPorts=2
  Scope4 : Scope  NumInputPorts=2
  Subsystem : Subsystem
  Subsystem1 : Subsystem
  Subsystem10 : Subsystem
  Subsystem11 : Subsystem
      mask Display: disp('Additional Load Meas.')
  Subsystem3 : Subsystem
  Subsystem4 : Subsystem
  Subsystem5 : Subsystem
  Subsystem6 : Subsystem
  Subsystem7 : Subsystem
  Subsystem8 : Subsystem
  Subsystem9 : Subsystem
  To Workspace : ToWorkspace  VariableName=t  SampleTime=5e-6
  wires:
  Product/1 -> PV Array Measurements/3, Subsystem4/1(Ppv)
  [Vpv] -> LPF vq2/1
  [Ipv_array] -> PV Array Measurements/2, Product/2
  [Irr] -> PV Array Measurements/4
  [SOC] -> Gain1/1
  [Ibat] -> Battery Measurements/2, Product4/1
  [Vbat] -> Battery Measurements/3, Product4/2
  Product4/1 -> Battery Measurements/4, Subsystem5/1(Pbat)
  [Vdc] -> LPF vq5/1
  [Idc] -> LPF vq4/1
  Product2/1 -> DC Bus Measurements BATTERY SIDE/3, Subsystem3/1(Pdc)
  Product1/1 -> DC Bus Measurements PV SIDE/3, Subsystem1/1(Pbus)
  [Vbus] -> LPF vq7/1
  [Ibus] -> LPF vq6/1
  Load Power Calculation/1(Pload) -> Load Powers/1
  Load Power Calculation/2(Qload) -> Load Powers/2
  [Vload_a] -> Scope11/1, RMS1/1
  RMS1/1 -> LPF1/1
  [Vload_ab] -> Scope4/1, RMS3/1
  RMS3/1 -> LPF/1
  LPF/1 -> Scope4/2, Subsystem6/1(Vab_rms)
  LPF1/1 -> Scope11/2, Subsystem7/1(Va_rms)
  Clock/1 -> To Workspace/1
  Product5/1 -> Subsystem8/1(Pdcinv), DC Bus Measurements INVERTER SIDE/3
  [Vdcinv] -> LPF vq3/1
  [Idcinv] -> LPF vq1/1
  LPF vq2/1 -> PV Array Measurements/1, Product/1
  LPF vq1/1 -> DC Bus Measurements INVERTER SIDE/2, Product5/2
  LPF vq3/1 -> DC Bus Measurements INVERTER SIDE/1, Product5/1
  LPF vq4/1 -> Product2/2, DC Bus Measurements BATTERY SIDE/2
  LPF vq5/1 -> Product2/1, DC Bus Measurements BATTERY SIDE/1
  LPF vq6/1 -> DC Bus Measurements PV SIDE/2, Product1/2
  LPF vq7/1 -> [A], DC Bus Measurements PV SIDE/1, Product1/1
  [w_abc] -> Gain/1
  Gain/1 -> Frequency/1, LPF vq10/1, Gain2/1
  LPF vq10/1 -> Frequency/2
  Subsystem9/1(Iabc) -> AC Load Measurements/2
  Subsystem/1(Vabc) -> Gain3/1
  Gain1/1 -> Battery Measurements/1
  Gain2/1 -> Subsystem10/1(f)
  Gain3/1 -> AC Load Measurements/1

== system microgrid/Subsystem1 ==
  Vdc_ref : Inport
  LPF vq6 : powerlib_extras/Discrete  Control Blocks/Discrete 1st-Order Filter  FilterType=Lowpass  Tc=10e-3  Ts=5e-6  Initialize=on  Vac_Init=[0.8 -25 60]  Vdc_Init=mg.Vbus_nom  PlotResponse=off  param1=[1 100 0.1]
      settings: SourceProductBaseCode=PS
  To Workspace1 : ToWorkspace  VariableName=Vdc_ref  SampleTime=-1
  tag scope: Vdc_ref=global
  wires:
  Vdc_ref/1 -> LPF vq6/1
  LPF vq6/1 -> [Vdc_ref], To Workspace1/1

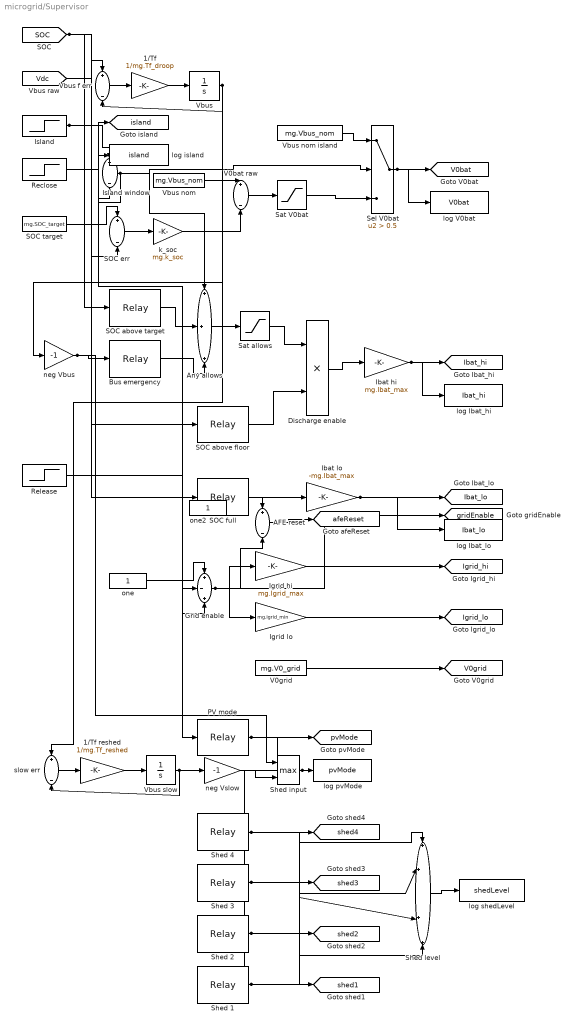
== system microgrid/Supervisor ==
  1/Tf : Gain  Gain=1/mg.Tf_droop
  1/Tf reshed : Gain  Gain=1/mg.Tf_reshed
  AFE reset : Sum  Inputs=+-
  Any allows : Sum  Inputs=+++
  Bus emergency : Relay  OnSwitchValue=-mg.Vbus_emerg  OffSwitchValue=-mg.Vbus_emerg_off
  Discharge enable : Product
  Grid enable : Sum  Inputs=+-+
  Ibat hi : Gain  Gain=mg.Ibat_max
  Ibat lo : Gain  Gain=-mg.Ibat_max
  Igrid hi : Gain  Gain=mg.Igrid_max
  Igrid lo : Gain  Gain=mg.Igrid_min
  Island : Step  Time=mg.t_island  SampleTime=0
  Island window : Sum  Inputs=+-
  PV mode : Relay  OnSwitchValue=mg.Vpv_ctrl_on  OffSwitchValue=mg.Vpv_ctrl_off  OnOutputValue=0  OffOutputValue=1
  Reclose : Step  Time=mg.t_reconnect  SampleTime=0
  Release : Step  Time=mg.t_reconnect+mg.t_resync  SampleTime=0
  SOC above floor : Relay  OnSwitchValue=mg.SOC_min+mg.SOC_hyst  OffSwitchValue=mg.SOC_min
  SOC above target : Relay  OnSwitchValue=mg.SOC_target+mg.SOC_hyst/2  OffSwitchValue=mg.SOC_target-mg.SOC_hyst/2
  SOC err : Sum  Inputs=+-
  SOC full : Relay  OnSwitchValue=mg.SOC_max  OffSwitchValue=mg.SOC_max-mg.SOC_hyst  OnOutputValue=0  OffOutputValue=1
  SOC target : Constant  Value=mg.SOC_target
  Sat V0bat : Saturate  UpperLimit=mg.V0bat_max  LowerLimit=mg.V0bat_min
  Sat allows : Saturate  UpperLimit=1  LowerLimit=0
  Sel V0bat : Switch  Criteria=u2 > Threshold  Threshold=0.5
  Shed 1 : Relay  OnSwitchValue=-mg.Vshed(4)  OffSwitchValue=-mg.Vshed_rst(4)
  Shed 2 : Relay  OnSwitchValue=-mg.Vshed(3)  OffSwitchValue=-mg.Vshed_rst(3)
  Shed 3 : Relay  OnSwitchValue=-mg.Vshed(2)  OffSwitchValue=-mg.Vshed_rst(2)
  Shed 4 : Relay  OnSwitchValue=-mg.Vshed(1)  OffSwitchValue=-mg.Vshed_rst(1)
  Shed input : MinMax  Function=max  Inputs=2
  Shed level : Sum  Inputs=++++
  V0bat raw : Sum  Inputs=+-
  V0grid : Constant  Value=mg.V0_grid
  Vbus : Integrator  InitialCondition=mg.Vbus_nom
  Vbus f err : Sum  Inputs=+-
  Vbus nom : Constant  Value=mg.Vbus_nom
  Vbus nom island : Constant  Value=mg.Vbus_nom
  Vbus slow : Integrator  InitialCondition=mg.Vbus_nom
  k_soc : Gain  Gain=mg.k_soc
  log Ibat_hi : ToWorkspace  VariableName=Ibat_hi  SaveFormat=Structure With Time  SampleTime=-1
      settings: Decimation=20
  log Ibat_lo : ToWorkspace  VariableName=Ibat_lo  SaveFormat=Structure With Time  SampleTime=-1
      settings: Decimation=20
  log V0bat : ToWorkspace  VariableName=V0bat  SaveFormat=Structure With Time  SampleTime=-1
      settings: Decimation=20
  log island : ToWorkspace  VariableName=island  SaveFormat=Structure With Time  SampleTime=-1
      settings: Decimation=20
  log pvMode : ToWorkspace  VariableName=pvMode  SaveFormat=Structure With Time  SampleTime=-1
      settings: Decimation=20
  log shedLevel : ToWorkspace  VariableName=shedLevel  SaveFormat=Structure With Time  SampleTime=-1
      settings: Decimation=20
  neg Vbus : Gain  Gain=-1
  neg Vslow : Gain  Gain=-1
  one : Constant
  one2 : Constant
  slow err : Sum  Inputs=+-
  tag scope: Ibat_hi=global, Ibat_lo=global, Igrid_hi=global, Igrid_lo=global, V0bat=global, V0grid=global, afeReset=global, gridEnable=global, island=global, pvMode=global, shed1=global, shed2=global, shed3=global, shed4=global
  wires:
  [Vdc] -> Vbus f err/1
  Vbus f err/1 -> 1/Tf/1
  1/Tf/1 -> Vbus/1
  Vbus/1 -> Vbus f err/2, neg Vbus/1, PV mode/1, slow err/1
  SOC target/1 -> SOC err/1
  [SOC] -> SOC err/2, SOC above target/1, SOC above floor/1, SOC full/1
  SOC err/1 -> k_soc/1
  Vbus nom/1 -> V0bat raw/1
  k_soc/1 -> V0bat raw/2
  V0bat raw/1 -> Sat V0bat/1
  Vbus nom island/1 -> Sel V0bat/1
  Sat V0bat/1 -> Sel V0bat/3
  Sel V0bat/1 -> [V0bat], log V0bat/1
  neg Vbus/1 -> Bus emergency/1, Shed input/1
  SOC above target/1 -> Any allows/2
  Bus emergency/1 -> Any allows/3
  Any allows/1 -> Sat allows/1
  Sat allows/1 -> Discharge enable/1
  SOC above floor/1 -> Discharge enable/2
  Discharge enable/1 -> Ibat hi/1
  Ibat hi/1 -> [Ibat_hi], log Ibat_hi/1
  SOC full/1 -> Ibat lo/1
  Ibat lo/1 -> [Ibat_lo], log Ibat_lo/1
  one/1 -> Grid enable/1
  Grid enable/1 -> Igrid hi/1, Igrid lo/1, [gridEnable], AFE reset/2
  Igrid hi/1 -> [Igrid_hi]
  Igrid lo/1 -> [Igrid_lo]
  V0grid/1 -> [V0grid]
  PV mode/1 -> [pvMode], log pvMode/1
  Island/1 -> Grid enable/2, Island window/1
  Reclose/1 -> Island window/2
  Island window/1 -> Sel V0bat/2, Any allows/1, [island], log island/1
  Release/1 -> Grid enable/3
  one2/1 -> AFE reset/1
  AFE reset/1 -> [afeReset]
  Shed 4/1 -> [shed4], Shed level/4
  Shed 3/1 -> [shed3], Shed level/3
  Shed 2/1 -> [shed2], Shed level/2
  Shed 1/1 -> [shed1], Shed level/1
  Shed level/1 -> log shedLevel/1
  slow err/1 -> 1/Tf reshed/1
  1/Tf reshed/1 -> Vbus slow/1
  Vbus slow/1 -> slow err/2, neg Vslow/1
  neg Vslow/1 -> Shed input/2
  Shed input/1 -> Shed 1/1, Shed 2/1, Shed 3/1, Shed 4/1

== system microgrid/Battery/Subsystem1 ==
  Ibat : Inport
  To Workspace1 : ToWorkspace  VariableName=Ibat  SampleTime=-1
  tag scope: Ibat=global
  wires:
  Ibat/1 -> To Workspace1/1, [Ibat]

== system microgrid/Battery/Subsystem2 ==
  Vbat : Inport
  To Workspace1 : ToWorkspace  VariableName=Vbat  SampleTime=-1
  tag scope: Vbat=global
  wires:
  Vbat/1 -> To Workspace1/1, [Vbat]

== system microgrid/Battery/Subsystem5 ==
  SOC : Inport
  To Workspace1 : ToWorkspace  VariableName=SOC  SampleTime=-1
  tag scope: SOC=global
  wires:
  SOC/1 -> To Workspace1/1, [SOC]

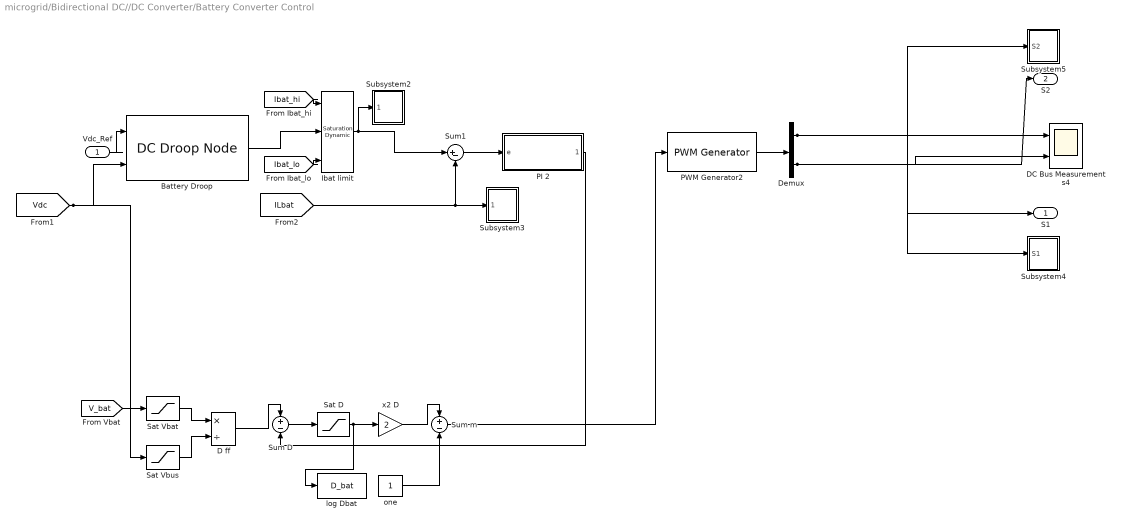
== system microgrid/Bidirectional DC//DC Converter/Battery Converter Control ==
  Vdc_Ref : Inport
  Battery Droop : microgridLib/DC Droop Node  Rdroop=mg.Rdroop_bat  DB=mg.DB_bat  Tf=mg.Tf_droop  Imin=-mg.Ibat_max  Imax=mg.Ibat_max  Vinit=mg.Vbus_nom
  D ff : Product  Inputs=*/
  DC Bus Measurements4 : Scope  NumInputPorts=2
  Demux : Demux  Outputs=2
  Ibat limit : simulink/Discontinuities/Saturation Dynamic  OutMin=[]  OutMax=[]  OutDataTypeStr=Inherit: Same as second input  OutDataType=fixdt(1, 16)  OutScaling=2^-10  DoSatur=off
  PI 2 : Subsystem
  PWM Generator2 : powerlib_extras/Control  Blocks/PWM Generator  GeneratorMode="1-arm  bridge (2 pulses)"  Fc=mg.fsw_bat  Internal=off  mIndex=0.4  Freq=mg.fgrid  Phase=0
      settings: SourceProductBaseCode=PS
  Sat D : Saturate  UpperLimit=mg.Dbat_max  LowerLimit=mg.Dbat_min
  Sat Vbat : Saturate  UpperLimit=inf  LowerLimit=mg.Vbat_ff_min
  Sat Vbus : Saturate  UpperLimit=inf  LowerLimit=mg.Vbus_ff_min
  Subsystem2 : Subsystem
  Subsystem3 : Subsystem
  Subsystem4 : Subsystem
  Subsystem5 : Subsystem
  Sum D : Sum  Inputs=+-
  Sum m : Sum  Inputs=+-
  Sum1 : Sum  Inputs=|+-
  log Dbat : ToWorkspace  VariableName=D_bat  SampleTime=-1
      settings: Decimation=20
  one : Constant
  x2 D : Gain  Gain=2
  S1 : Outport
  S2 : Outport  Port=2
  wires:
  Sum1/1 -> PI 2/1(e)
  [ILbat] -> Sum1/2, Subsystem3/1(ILbat)
  [Vdc] -> Sat Vbus/1, Battery Droop/2
  [V_bat] -> Sat Vbat/1
  Sat Vbat/1 -> D ff/1
  Sat Vbus/1 -> D ff/2
  D ff/1 -> Sum D/1
  PI 2/1(" ") -> Sum D/2
  Sat D/1 -> x2 D/1, log Dbat/1
  x2 D/1 -> Sum m/1
  one/1 -> Sum m/2
  Sum D/1 -> Sat D/1
  Sum m/1 -> PWM Generator2/1
  PWM Generator2/1 -> Demux/1
  Demux/1 -> S1/1, Subsystem4/1(S1), DC Bus Measurements4/1
  Demux/2 -> S2/1, Subsystem5/1(S2), DC Bus Measurements4/2
  Vdc_Ref/1 -> Battery Droop/1
  [Ibat_hi] -> Ibat limit/1
  Battery Droop/1 -> Ibat limit/2
  [Ibat_lo] -> Ibat limit/3
  Ibat limit/1 -> Subsystem2/1(Ibat_ref), Sum1/1

== system microgrid/Bidirectional DC//DC Converter/Subsystem1 ==
  Idc : Inport
  LPF vq11 : powerlib_extras/Discrete  Control Blocks/Discrete 1st-Order Filter  FilterType=Lowpass  Tc=10e-3  Ts=5e-6  Initialize=off  Vac_Init=[0.8 -25 60]  Vdc_Init=0  PlotResponse=off  param1=[1 100 0.1]
      settings: SourceProductBaseCode=PS
  To Workspace1 : ToWorkspace  VariableName=Idc  SampleTime=-1
  To Workspace2 : ToWorkspace  VariableName=Idc1  SampleTime=-1
  tag scope: Idc=global
  wires:
  Idc/1 -> [Idc], To Workspace1/1, LPF vq11/1
  LPF vq11/1 -> To Workspace2/1

== system microgrid/Bidirectional DC//DC Converter/Subsystem2 ==
  Vdc : Inport
  LPF vq11 : powerlib_extras/Discrete  Control Blocks/Discrete 1st-Order Filter  FilterType=Lowpass  Tc=10e-3  Ts=5e-6  Initialize=off  Vac_Init=[0.8 -25 60]  Vdc_Init=0  PlotResponse=off  param1=[1 100 0.1]
      settings: SourceProductBaseCode=PS
  To Workspace1 : ToWorkspace  VariableName=Vdc  SampleTime=-1
  To Workspace2 : ToWorkspace  VariableName=Vdc1  SampleTime=-1
  tag scope: Vdc=global
  wires:
  Vdc/1 -> [Vdc], To Workspace1/1, LPF vq11/1
  LPF vq11/1 -> To Workspace2/1
